simulink model "Exp4_2"  (R2024a)
settings: Solver=ode1  StartTime=0.0  StopTime=10.0  FixedStep=1e-3  RelTol=1e-3
settings Model: Creator=Rodrigo  LastModifiedBy=Rodrigo

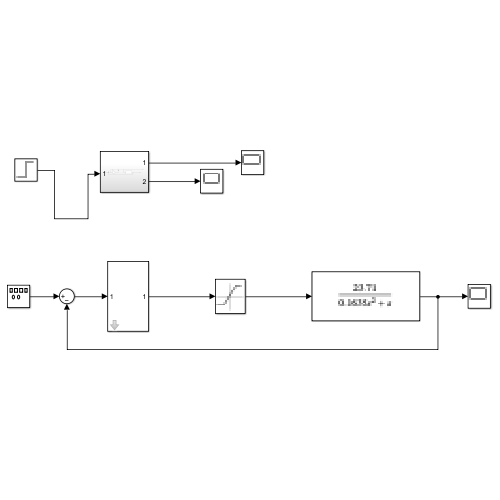
[thumbnail: Simulink's stored preview of the top-level diagram]
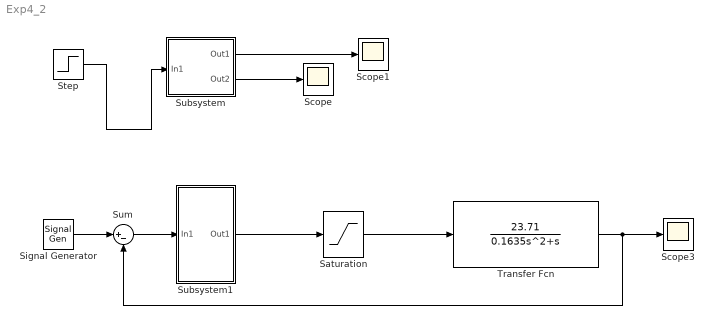
== system Exp4_2 ==
  Saturation : Saturate  UpperLimit=10  LowerLimit=-10
  Scope : Scope
  Scope1 : Scope
  Scope3 : Scope
  Signal Generator : SignalGenerator  WaveForm=square  Amplitude=2  Frequency=.1
  Step : Step  After=0.8  SampleTime=0
  Subsystem : Subsystem
  Subsystem1 : Subsystem  mask{KP=12.3, KD=0.25, KI=0, tau=0.1635, Umax=10, Umin=-10}
  Sum : Sum  Inputs=|+-
  Transfer Fcn : TransferFcn  Numerator=[23.71]  Denominator=[0.1635 1 0]
  wires:
  Step/1 -> Subsystem/1(In1)
  Subsystem/1(Out1) -> Scope1/1
  Subsystem/2(Out2) -> Scope/1
  Subsystem1/1(Out1) -> Saturation/1
  Saturation/1 -> Transfer Fcn/1
  Transfer Fcn/1 -> Scope3/1, Sum/2
  Sum/1 -> Subsystem1/1(In1)
  Signal Generator/1 -> Sum/1

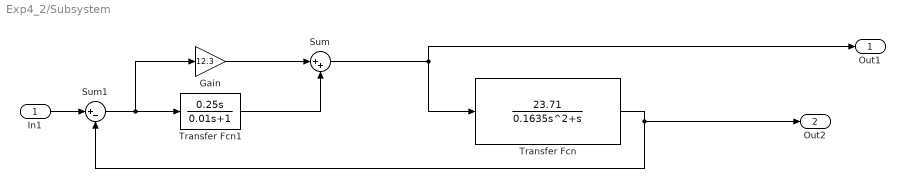
== system Exp4_2/Subsystem ==
  In1 : Inport
  Gain : Gain  Gain=12.3
  Sum : Sum  Inputs=|++
  Sum1 : Sum  Inputs=|+-
  Transfer Fcn : TransferFcn  Numerator=[23.71]  Denominator=[0.1635 1 0]
  Transfer Fcn1 : TransferFcn  Numerator=[0.25 0]  Denominator=[0.01 1]
  Out1 : Outport
  Out2 : Outport  Port=2
  wires:
  Sum1/1 -> Gain/1, Transfer Fcn1/1
  Transfer Fcn1/1 -> Sum/2
  Transfer Fcn/1 -> Out2/1, Sum1/2
  Gain/1 -> Sum/1
  Sum/1 -> Out1/1, Transfer Fcn/1
  In1/1 -> Sum1/1

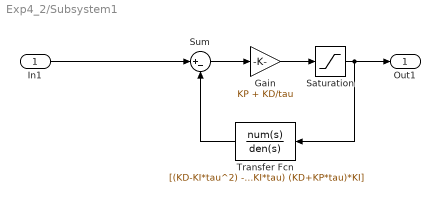
== system Exp4_2/Subsystem1 ==
  In1 : Inport
  Gain : Gain  Gain=KP + KD/tau
  Saturation : Saturate  UpperLimit=Umax  LowerLimit=Umin
  Sum : Sum  Inputs=|+-
  Transfer Fcn : TransferFcn  Numerator=[(KD-KI*tau^2) -(tau*KI)]  Denominator=[(KD+KP*tau)^2 (KD+KP*tau)*(KP+KI*tau) (KD+KP*tau)*KI]
  Out1 : Outport
  wires:
  In1/1 -> Sum/1
  Saturation/1 -> Out1/1, Transfer Fcn/1
  Gain/1 -> Saturation/1
  Sum/1 -> Gain/1
  Transfer Fcn/1 -> Sum/2
